simulink model "controladorARX"  (R2023b)
settings: Solver=VariableStepAuto  StartTime=0.0  StopTime=0.008  RelTol=1e-3
undefined symbols (not defined in the file): denS, gainI, gainP, numS
settings Model: Creator=luisf  LastModifiedBy=luisf

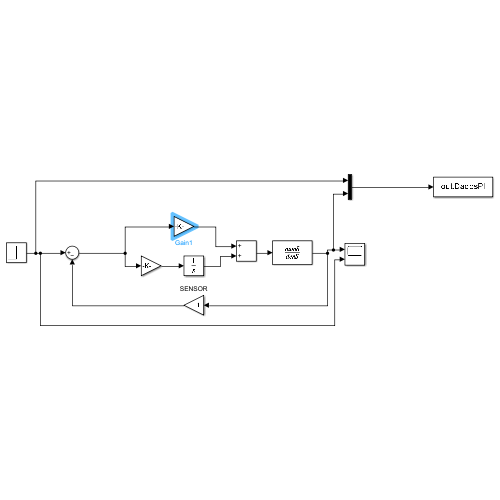
[thumbnail: Simulink's stored preview of the top-level diagram]
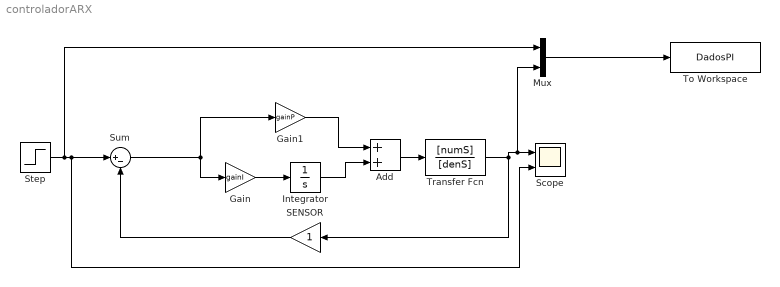
== system controladorARX ==
  Add : Sum
  Gain : Gain  Gain=gainI
  Gain1 : Gain  Gain=gainP
  Integrator : Integrator
  Mux : Mux  Inputs=2
  SENSOR : Gain
  Scope : Scope  NumInputPorts=2
  Step : Step  Time=0.001  SampleTime=0
  Sum : Sum  Inputs=|+-
  To Workspace : ToWorkspace  VariableName=DadosPI  SampleTime=-1
  Transfer Fcn : TransferFcn  Numerator=[numS]  Denominator=[denS]
  wires:
  Gain1/1 -> Add/1
  Mux/1 -> To Workspace/1
  SENSOR/1 -> Sum/2
  Transfer Fcn/1 -> SENSOR/1, Mux/2, Scope/1
  Add/1 -> Transfer Fcn/1
  Integrator/1 -> Add/2
  Sum/1 -> Gain1/1, Gain/1
  Gain/1 -> Integrator/1
  Step/1 -> Mux/1, Scope/2, Sum/1
